simulink model "FamlyRStateCtrl"  (R2018b)
settings: Solver=FixedStepDiscrete  StartTime=0.0  StopTime=10.0  FixedStep=0.01  RelTol=1e-3
libraries: StateCtrlLib x1
settings Model: Creator=sn2xws  LastModifiedBy=sn2xws
settings DataIOCC: SaveFormat=StructureWithTime
settings OptimizationCC: DefaultParameterBehavior=Inlined  EnhancedBackFolding=on  PassReuseOutputArgsAs=Individual arguments  ZeroExternalMemoryAtStartup=off  ZeroInternalMemoryAtStartup=off  OptimizeBlockOrder=speed  DifferentSizesBufferReuse=on  OptimizationCustomize=off
settings DebuggingCC: ParameterTunabilityLossMsg=error
settings ModelReferenceCC: ModelReferenceNumInstancesAllowed=Single
settings SFSimCC: MATLABDynamicMemAlloc=off
settings RTWCC: SystemTargetFile=autosar.tlc  GenCodeOnly=on  TemplateMakefile=ert_default_tmf  Description=AUTOSAR  GenerateReport=on  IncludeHyperlinkInReport=on  LaunchReport=on  GenerateTraceInfo=on  GenerateTraceReport=on  GenerateTraceReportSl=on  GenerateTraceReportSf=on  GenerateTraceReportEml=on
settings CodeAppCC: ForceParamTrailComments=on  IgnoreCustomStorageClasses=off  OperatorAnnotations=on  SimulinkDataObjDesc=on  SFDataObjDesc=on  InsertBlockDesc=on
settings STFCustomTargetCC: TargetLangStandard=C99 (ISO)  MultiwordLength=256  ParMdlRefBuildCompliant=on  CompOptLevelCompliant=on  IncludeMdlTerminateFcn=off  CombineOutputUpdateFcns=on  SuppressErrorStatus=on  ERTCustomFileBanners=on  SupportNonFinite=off  SupportComplex=off  SupportContinuousTime=off  SupportNonInlinedSFcns=off  RemoveResetFunc=on  MATLABClassNameForMDSCustomization=Simulink.SoftwareTarget.ERTCustomization  AutosarCompliant=on  UseToolchainInfoCompliant=on  LookupTableObjectStructAxisOrder=2,1,3,4,...  LUTObjectStructOrderEvenSpacing=Size,Table,Breakpoints  SystemTargetFile=autosar.tlc
settings ERTTargetCC: TargetLangStandard=C99 (ISO)  ConcurrentExecutionCompliant=off  IncludeMdlTerminateFcn=off  SuppressErrorStatus=on  SupportNonFinite=off  SupportComplex=off  ModelStepFunctionPrototypeControlCompliant=off  CPPClassGenCompliant=off  AutosarCompliant=on  LookupTableObjectStructAxisOrder=2,1,3,4,...  LUTObjectStructOrderEvenSpacing=Size,Table,Breakpoints  InlinedParameterPlacement=NonHierarchical  ERTCustomFileTemplate=example_file_process.tlc

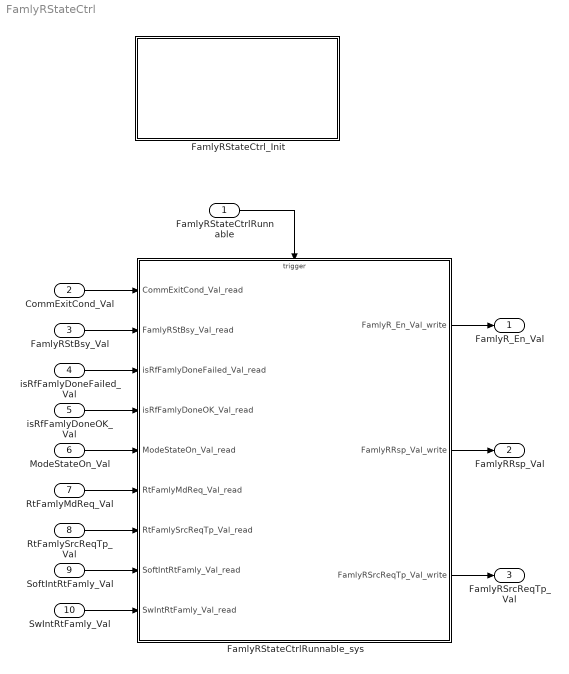
== system FamlyRStateCtrl ==
  FamlyRStateCtrlRunnable : Inport  SampleTime=0.01  OutputFunctionCall=on
  CommExitCond_Val : Inport  Port=2  OutDataTypeStr=boolean  PortDimensions=1
  FamlyRStBsy_Val : Inport  Port=3  OutDataTypeStr=boolean  PortDimensions=1
  isRfFamlyDoneFailed_Val : Inport  Port=4  OutDataTypeStr=boolean  PortDimensions=1
  isRfFamlyDoneOK_Val : Inport  Port=5  OutDataTypeStr=boolean  PortDimensions=1
  ModeStateOn_Val : Inport  Port=6  OutDataTypeStr=boolean  PortDimensions=1
  RtFamlyMdReq_Val : Inport  Port=7  OutDataTypeStr=boolean  PortDimensions=1
  RtFamlySrcReqTp_Val : Inport  Port=8  OutDataTypeStr=Enum: SrcReqTp1  PortDimensions=1
  SoftIntRtFamly_Val : Inport  Port=9  OutDataTypeStr=IntEnable  PortDimensions=1
  SwIntRtFamly_Val : Inport  Port=10  OutDataTypeStr=IntEnable  PortDimensions=1
  FamlyRStateCtrlRunnable_sys : Subsystem
  FamlyRStateCtrl_Init : Subsystem
  FamlyR_En_Val : Outport  OutDataTypeStr=boolean  PortDimensions=1
  FamlyRRsp_Val : Outport  Port=2  OutDataTypeStr=Enum: MdRspLocal1  PortDimensions=1
  FamlyRSrcReqTp_Val : Outport  Port=3  OutDataTypeStr=Enum: SrcReqTp1  PortDimensions=1
  wires:
  CommExitCond_Val/1 -> FamlyRStateCtrlRunnable_sys/1(CommExitCond_Val_read)
  FamlyRStBsy_Val/1 -> FamlyRStateCtrlRunnable_sys/2(FamlyRStBsy_Val_read)
  isRfFamlyDoneFailed_Val/1 -> FamlyRStateCtrlRunnable_sys/3(isRfFamlyDoneFailed_Val_read)
  isRfFamlyDoneOK_Val/1 -> FamlyRStateCtrlRunnable_sys/4(isRfFamlyDoneOK_Val_read)
  ModeStateOn_Val/1 -> FamlyRStateCtrlRunnable_sys/5(ModeStateOn_Val_read)
  RtFamlyMdReq_Val/1 -> FamlyRStateCtrlRunnable_sys/6(RtFamlyMdReq_Val_read)
  RtFamlySrcReqTp_Val/1 -> FamlyRStateCtrlRunnable_sys/7(RtFamlySrcReqTp_Val_read)
  SoftIntRtFamly_Val/1 -> FamlyRStateCtrlRunnable_sys/8(SoftIntRtFamly_Val_read)
  SwIntRtFamly_Val/1 -> FamlyRStateCtrlRunnable_sys/9(SwIntRtFamly_Val_read)
  FamlyRStateCtrlRunnable_sys/1(FamlyR_En_Val_write) -> FamlyR_En_Val/1
  FamlyRStateCtrlRunnable_sys/2(FamlyRRsp_Val_write) -> FamlyRRsp_Val/1
  FamlyRStateCtrlRunnable_sys/3(FamlyRSrcReqTp_Val_write) -> FamlyRSrcReqTp_Val/1
  FamlyRStateCtrlRunnable/1 -> FamlyRStateCtrlRunnable_sys/Trigger

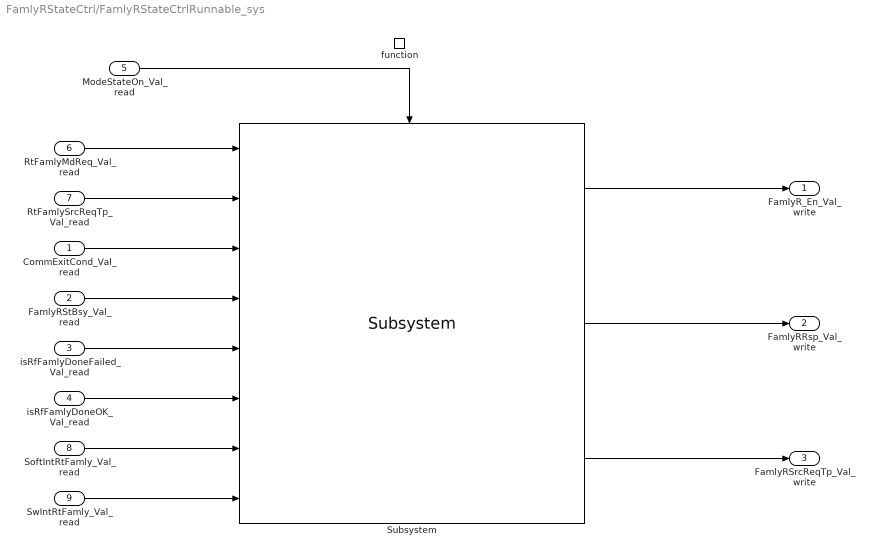
== system FamlyRStateCtrl/FamlyRStateCtrlRunnable_sys ==
  CommExitCond_Val_read : Inport
  FamlyRStBsy_Val_read : Inport  Port=2
  isRfFamlyDoneFailed_Val_read : Inport  Port=3
  isRfFamlyDoneOK_Val_read : Inport  Port=4
  ModeStateOn_Val_read : Inport  Port=5
  RtFamlyMdReq_Val_read : Inport  Port=6
  RtFamlySrcReqTp_Val_read : Inport  Port=7
  SoftIntRtFamly_Val_read : Inport  Port=8  OutDataTypeStr=IntEnable
  SwIntRtFamly_Val_read : Inport  Port=9  OutDataTypeStr=IntEnable
  function : TriggerPort  TriggerType=function-call  VariantControl=(inherit)  SampleTimeType=periodic  SampleTime=-1
  Subsystem : StateCtrlLib/Subsystem  SystemSampleTime=-1
  FamlyR_En_Val_write : Outport
      settings: EnsureOutportIsVirtual=on
  FamlyRRsp_Val_write : Outport  Port=2
      settings: EnsureOutportIsVirtual=on
  FamlyRSrcReqTp_Val_write : Outport  Port=3
      settings: EnsureOutportIsVirtual=on
  wires:
  ModeStateOn_Val_read/1 -> Subsystem/Enable
  SoftIntRtFamly_Val_read/1 -> Subsystem/7
  SwIntRtFamly_Val_read/1 -> Subsystem/8
  Subsystem/1 -> FamlyR_En_Val_write/1
  Subsystem/2 -> FamlyRRsp_Val_write/1
  Subsystem/3 -> FamlyRSrcReqTp_Val_write/1
  RtFamlyMdReq_Val_read/1 -> Subsystem/1
  RtFamlySrcReqTp_Val_read/1 -> Subsystem/2
  CommExitCond_Val_read/1 -> Subsystem/3
  FamlyRStBsy_Val_read/1 -> Subsystem/4
  isRfFamlyDoneFailed_Val_read/1 -> Subsystem/5
  isRfFamlyDoneOK_Val_read/1 -> Subsystem/6

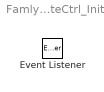
== system FamlyRStateCtrl/FamlyRStateCtrl_Init ==
  Event Listener : EventListener  EventName=reset
